simulink model "sinwave"  (R2016a)
settings: Solver=VariableStepAuto  StartTime=0.0  StopTime=10.0  RelTol=1e-3
settings Model: Creator=areej_ofamech  LastModifiedBy=areej_ofamech
settings GRTTargetCC: GeneratePreprocessorConditionals=Use local settings

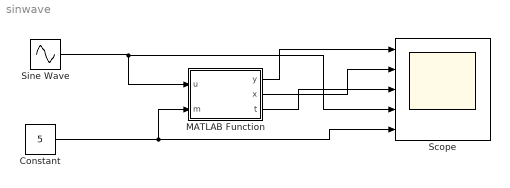
== system sinwave ==
  Constant : Constant  Value=5
  MATLAB Function : MATLAB Function  TreatAsAtomicUnit=on
  Scope : Scope  NumInputPorts=5
  Sine Wave : Sin  SampleTime=0
  wires:
  Sine Wave/1 -> Scope/4, MATLAB Function/1(u)
  Constant/1 -> Scope/5, MATLAB Function/2(m)
  MATLAB Function/1(y) -> Scope/1
  MATLAB Function/2(x) -> Scope/2
  MATLAB Function/3(t) -> Scope/3

== matlab function sinwave/MATLAB Function ==
  data: u input; y output; x output; m input; t output
function [y,x,t] = fcn(u,m)
%#codegen

y = u+m;
x=u*m;
t=y-u;
